simulink model "ESCHighLevelSim"  (R2021b)
settings: Solver=FixedStepDiscrete  StartTime=0.0  StopTime=15  FixedStep=0.008  RelTol=1e-3
InitFcn:
  | ts = 0.008
  | ESCHighLevelInit
values from neighbouring files (symbols this model uses):
  AbsActSpdThre = 10/3.6    (= 2.77777777778)    [ESCHighLevelInit.m]
  AbsBrkChkThre = 0.8    [ESCHighLevelInit.m]
  AbsCriDelay = 4    [ESCHighLevelInit.m]
  AbsLockJudgeThre = 0.006    [ESCHighLevelInit.m]
  AbsLockSlipThre1 = 0.05    [ESCHighLevelInit.m]
  AbsLockSlipThre2 = 0.15    [ESCHighLevelInit.m]
  AbsSpdEstRelayT = 40    [ESCHighLevelInit.m]
  FrontAngleDeadZone = 0.5*3.14/180    (= 0.00872222222222)    [ESCHighLevelInit.m]
  VehParaD = 1.958    [ESCHighLevelInit.m]
  VehParaL = 4.39    [ESCHighLevelInit.m]
  VehParaR = 0.376    [ESCHighLevelInit.m]
undefined symbols (not defined in the file or in its folder): Discrete, Time, VehR
libraries: dspstat3 x7, simulink x5, ctrlSharedLib x1
settings Model: Creator=Huiqian  LastModifiedBy=Huiqian
settings OptimizationCC: DefaultParameterBehavior=Inlined  UseDivisionForNetSlopeComputation=on  GainParamInheritBuiltInType=on  UseFloatMulNetSlope=on  InlineInvariantSignals=on  PassReuseOutputArgsAs=Individual arguments  ZeroExternalMemoryAtStartup=off  ZeroInternalMemoryAtStartup=off  NoFixptDivByZeroProtection=on  EfficientFloat2IntCast=on  LifeSpan=1  OptimizeBlockOrder=speed  DifferentSizesBufferReuse=on  EfficientTunableParamExpr=on
settings DebuggingCC: ParameterTunabilityLossMsg=error
settings HardwareCC: ProdBitPerPointer=32  ProdBitPerSizeT=32  ProdBitPerPtrDiffT=32  ProdLargestAtomicInteger=Long  ProdLargestAtomicFloat=Double  ProdWordSize=32  ProdLongLongMode=on  ProdHWDeviceType=NXP->Cortex-M4
settings SFSimCC: MATLABDynamicMemAlloc=off
settings RTWCC: Description=Embedded Coder  SystemTargetFile=ert.tlc  TemplateMakefile=ert_default_tmf  GenerateReport=on  LaunchReport=on
settings CodeAppCC: ForceParamTrailComments=on  IgnoreCustomStorageClasses=off  OperatorAnnotations=on  SimulinkDataObjDesc=on  SFDataObjDesc=on  CustomSymbolStrGlobalVar=rt$N$M  CustomSymbolStrType=$N$M  CustomSymbolStrFcn=$N$M$F  CustomSymbolStrMacro=$N$M  InsertBlockDesc=on
settings ERTTargetCC: TargetLangStandard=C99 (ISO)  GenerateSampleERTMain=on  IncludeMdlTerminateFcn=off  CombineSignalStateStructs=on  CodeInterfacePackaging=Reusable function  SupportComplex=off  SupportContinuousTime=on  SupportNonInlinedSFcns=on  InlinedParameterPlacement=NonHierarchical  ERTCustomFileTemplate=example_file_process.tlc

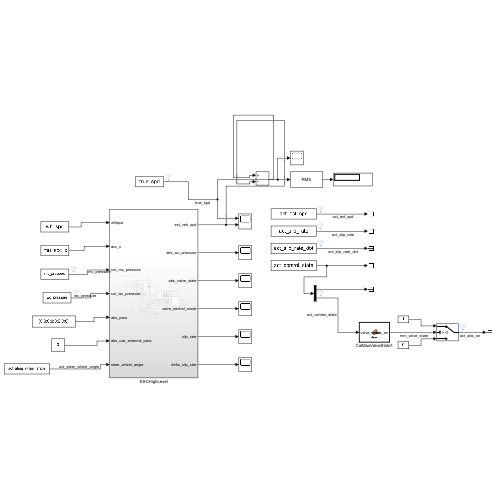
[thumbnail: Simulink's stored preview of the top-level diagram]
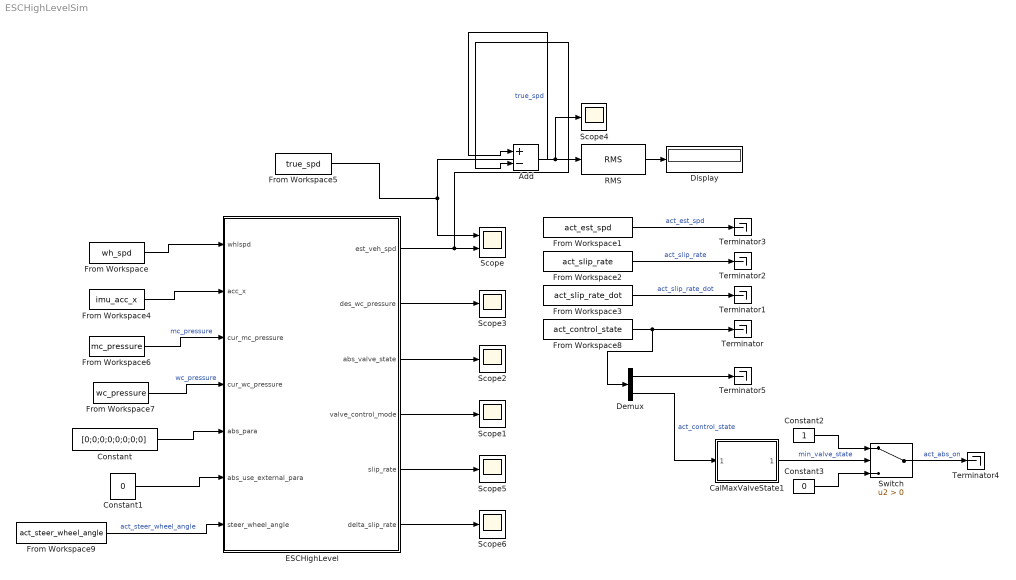
== system ESCHighLevelSim ==
  Add : Sum  Inputs=+-
  CalMaxValveState1 : MATLAB Function  TreatAsAtomicUnit=on
  Constant : Constant  Value=[0;0;0;0;0;0;0;0]  OutDataTypeStr=single
  Constant1 : Constant  Value=0  OutDataTypeStr=int32
  Constant2 : Constant  OutDataTypeStr=boolean
  Constant3 : Constant  Value=0  OutDataTypeStr=fixdt(1,16)
  Demux : Demux  Outputs=[2,4]
  Display : Display
  ESCHighLevel : Subsystem
  From Workspace : FromWorkspace  VariableName=wh_spd
  From Workspace1 : FromWorkspace  VariableName=act_est_spd
  From Workspace2 : FromWorkspace  VariableName=act_slip_rate
  From Workspace3 : FromWorkspace  VariableName=act_slip_rate_dot
  From Workspace4 : FromWorkspace  VariableName=imu_acc_x
  From Workspace5 : FromWorkspace  VariableName=true_spd
  From Workspace6 : FromWorkspace  VariableName=mc_pressure
  From Workspace7 : FromWorkspace  VariableName=wc_pressure
  From Workspace8 : FromWorkspace  VariableName=act_control_state
  From Workspace9 : FromWorkspace  VariableName=act_steer_wheel_angle
  RMS : dspstat3/RMS  run=off  directionMode=Each column  dimension=1  InputProcessing=Columns as channels (frame based)  reset_popup=None
  Scope : Scope  NumInputPorts=2
  Scope{1..6} (6 alike) : Scope
  Switch : Switch  Criteria=u2 > Threshold
  Terminator{,1..5} (6 alike) : Terminator
  wires:
  From Workspace/1 -> ESCHighLevel/1(whlspd)
  From Workspace6/1 -> ESCHighLevel/3(cur_mc_pressure)  "mc_pressure"
  ESCHighLevel/1(est_veh_spd) -> Add/2, Scope/2
  ESCHighLevel/2(des_wc_pressure) -> Scope3/1
  From Workspace7/1 -> ESCHighLevel/4(cur_wc_pressure)  "wc_pressure"
  From Workspace5/1 -> Scope/1, Add/1  "true_spd"
  Add/1 -> Scope4/1, RMS/1
  RMS/1 -> Display/1
  From Workspace4/1 -> ESCHighLevel/2(acc_x)
  ESCHighLevel/4(valve_control_mode) -> Scope1/1
  ESCHighLevel/3(abs_valve_state) -> Scope2/1
  Constant/1 -> ESCHighLevel/5(abs_para)
  Constant1/1 -> ESCHighLevel/6(abs_use_external_para)
  ESCHighLevel/5(slip_rate) -> Scope5/1
  ESCHighLevel/6(delta_slip_rate) -> Scope6/1
  From Workspace8/1 -> Demux/1, Terminator/1
  From Workspace3/1 -> Terminator1/1  "act_slip_rate_dot"
  From Workspace1/1 -> Terminator3/1  "act_est_spd"
  From Workspace2/1 -> Terminator2/1  "act_slip_rate"
  Switch/1 -> Terminator4/1  "act_abs_on"
  CalMaxValveState1/1(abs_on) -> Switch/2  "min_valve_state"
  Constant3/1 -> Switch/3
  Constant2/1 -> Switch/1
  Demux/1 -> Terminator5/1
  Demux/2 -> CalMaxValveState1/1(valve_state)  "act_control_state"
  From Workspace9/1 -> ESCHighLevel/7(steer_wheel_angle)  "act_steer_wheel_angle"

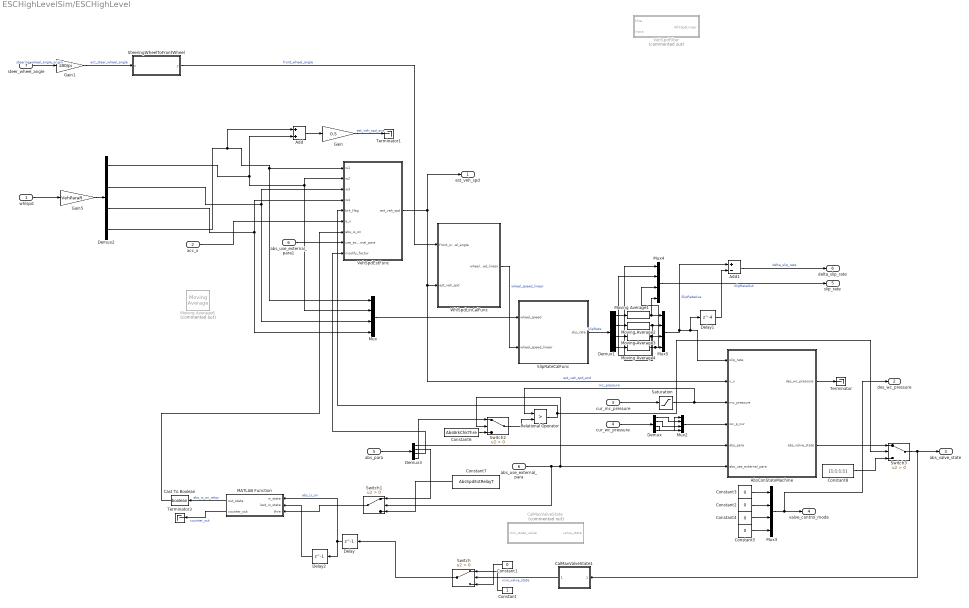
== system ESCHighLevelSim/ESCHighLevel ==
  whlspd : Inport  OutDataTypeStr=double  Unit=rad/s  PortDimensions=4
  acc_x : Inport  Port=2  OutDataTypeStr=double  Unit=m/s^2  PortDimensions=1
  cur_mc_pressure : Inport  Port=3  OutDataTypeStr=double  PortDimensions=1
  cur_wc_pressure : Inport  Port=4  OutDataTypeStr=double  PortDimensions=4
  abs_para : Inport  Port=5  OutDataTypeStr=single  PortDimensions=8
  abs_use_external_para : Inport  Port=6  OutDataTypeStr=int32  PortDimensions=1
  steer_wheel_angle : Inport  Port=7
  AbsConStateMachine : Subsystem  SystemSampleTime=0.01
      settings: MinAlgLoopOccurrences=on  RTWFcnNameOpts=Use subsystem name  RTWFileNameOpts=Use subsystem name
  Add : Sum
  Add1 : Sum  Inputs=+-
  CalMaxValveState : MATLAB Function  Commented=on  TreatAsAtomicUnit=on
  CalMaxValveState1 : MATLAB Function  TreatAsAtomicUnit=on
  Cast To Boolean : DataTypeConversion  OutDataTypeStr=boolean
  Constant : Constant  OutDataTypeStr=boolean
  Constant1 : Constant  Value=0  OutDataTypeStr=fixdt(1,16)
  Constant{2..5} (4 alike) : Constant  Value=0  OutDataTypeStr=int32
  Constant6 : Constant  Value=AbsBrkChkThre
  Constant7 : Constant  Value=AbsSpdEstRelayT
  Constant8 : Constant  Value=[1;1;1;1]
  Delay : Delay  DelayLength=1
  Delay1 : Delay  DelayLength=4
  Delay2 : Delay  DelayLength=1
  Demux : Demux
  Demux1 : Demux
  Demux2 : Demux
  Demux3 : Demux  Outputs=[5,1,1,1]
  Gain : Gain  Gain=0.5
  Gain1 : Gain  Gain=180/pi
  Gain5 : Gain  Gain=VehParaR
  MATLAB Function : MATLAB Function  TreatAsAtomicUnit=on
  Moving Average{1..4} (4 alike) : dspstat3/Moving Average  Method=Sliding window  ForgettingFactorPort=off  SpecifyWindowLength=on  WindowLength=3  ForgettingFactor=0.9  SimulateUsing=Code generation
  Moving Average6 : dspstat3/Moving Average  Commented=on  Method=Sliding window  ForgettingFactorPort=off  SpecifyWindowLength=on  WindowLength=5  ForgettingFactor=0.9  SimulateUsing=Code generation
  Mux{,2..5} (5 alike) : Mux
  Relational Operator : RelationalOperator  Operator=>  OutDataTypeStr=boolean  RndMeth=Simplest
  Saturation : Saturate  UpperLimit=10
  SlipRateCalFunc : Subsystem  TreatAsAtomicUnit=on
      settings: RTWFcnNameOpts=Use subsystem name  RTWFileNameOpts=Use subsystem name
  SteeringWheelToFrontWheel : MATLAB Function  TreatAsAtomicUnit=on
  Switch{,1..3} (4 alike) : Switch  Criteria=u2 > Threshold
  Terminator : Terminator
  Terminator1 : Terminator
  Terminator3 : Terminator
  VehSpdEstFunc : Subsystem  TreatAsAtomicUnit=on  SystemSampleTime=ts  RTWFcnName=VehSpdEstFunction  RTWFileName=VehSpdEstFunction
      settings: RTWFcnNameOpts=User specified  RTWFileNameOpts=User specified
  VehSpdFilter : Subsystem  Commented=on  TreatAsAtomicUnit=on
  WhlSpdLinCalFunc : Subsystem
  abs_use_external_para1 : InportShadow  Port=6  OutDataTypeStr=int32  PortDimensions=1
  est_veh_spd : Outport  OutDataTypeStr=double  Unit=m/s  PortDimensions=1
  des_wc_pressure : Outport  Port=2  PortDimensions=4
  abs_valve_state : Outport  Port=3  OutDataTypeStr=int32  PortDimensions=4
  valve_control_mode : Outport  Port=4  OutDataTypeStr=int32
  slip_rate : Outport  Port=5  OutDataTypeStr=double
  delta_slip_rate : Outport  Port=6  OutDataTypeStr=double
  wires:
  Demux3/4 -> Switch2/1
  Constant6/1 -> Switch2/3
  AbsConStateMachine/2(abs_valve_state) -> Switch3/1
  Switch3/1 -> abs_valve_state/1, CalMaxValveState1/1(valve_state)
  Constant8/1 -> Switch3/3
  Demux/3 -> Mux2/4
  Delay1/1 -> Add1/2
  Constant5/1 -> Mux3/4
  Demux/2 -> Mux2/3
  AbsConStateMachine/1(des_wc_pressure) -> Terminator/1
  Saturation/1 -> Relational Operator/1, AbsConStateMachine/3(mc_pressure)  "mc_pressure"
  Demux1/4 -> Moving Average4/1
  SlipRateCalFunc/1(slip_rate) -> Demux1/1  "SlipRate"
  Gain5/1 -> Demux2/1
  Switch1/1 -> MATLAB Function/3(thre)
  Demux1/1 -> Moving Average1/1
  Constant7/1 -> Switch1/3
  Demux3/2 -> Switch1/1
  Demux3/1 -> AbsConStateMachine/5(abs_para)
  Switch/1 -> Delay/1
  abs_para/1 -> Demux3/1
  Delay2/1 -> MATLAB Function/2(last_in_state)
  CalMaxValveState1/1(abs_on) -> Switch/2  "min_valve_state"
  Constant/1 -> Switch/1
  Add1/1 -> delta_slip_rate/1  "delta_slip_rate"
  cur_wc_pressure/1 -> Demux/1
  cur_mc_pressure/1 -> Saturation/1
  WhlSpdLinCalFunc/1(wheel_speed_linear) -> SlipRateCalFunc/2(wheel_speed_linear)  "wheel_speed_linear"
  Gain/1 -> Terminator1/1  "est_veh_spd_ave"
  MATLAB Function/2(counter_out) -> Terminator3/1  "counter_out"
  MATLAB Function/1(out_state) -> Cast To Boolean/1  "abs_is_on_relay"
  Moving Average2/1 -> Mux4/1, Mux5/2
  Mux/1 -> SlipRateCalFunc/1(wheel_speed)
  Switch2/1 -> Relational Operator/2
  Cast To Boolean/1 -> VehSpdEstFunc/7(abs_is_on)
  Demux3/3 -> VehSpdEstFunc/9(modify_factor)
  SteeringWheelToFrontWheel/1(y) -> WhlSpdLinCalFunc/1(front_wheel_angle)  "front_wheel_angle"
  Delay/1 -> Delay2/1, MATLAB Function/1(in_state)  "abs_is_on"
  steer_wheel_angle/1 -> Gain1/1  "steering_wheel_angle_origin"
  whlspd/1 -> Gain5/1
  Demux2/4 -> Add/1, Mux/1, VehSpdEstFunc/1(w1)
  Relational Operator/1 -> Switch3/2, VehSpdEstFunc/5(brk_flag)
  Demux1/3 -> Moving Average3/1
  Demux2/2 -> Mux/3, VehSpdEstFunc/3(w3)
  acc_x/1 -> VehSpdEstFunc/6(a_x)
  Demux2/1 -> Mux/2, VehSpdEstFunc/2(w2), Add/2
  abs_use_external_para/1 -> Switch1/2, Switch2/2, AbsConStateMachine/6(abs_use_external_para)
  Mux5/1 -> Add1/1, Delay1/1, AbsConStateMachine/1(slip_rate)  "SlipRateAve"
  Moving Average3/1 -> Mux5/3, Mux4/2
  Gain1/1 -> SteeringWheelToFrontWheel/1(x)  "act_steer_wheel_angle"
  Mux3/1 -> des_wc_pressure/1, valve_control_mode/1
  Demux/1 -> Mux2/2
  Constant1/1 -> Switch/3
  VehSpdEstFunc/1(est_veh_spd) -> est_veh_spd/1, WhlSpdLinCalFunc/2(est_veh_spd), AbsConStateMachine/2(v_x)  "est_veh_spd_end"
  Mux4/1 -> slip_rate/1  "SlipRateOut"
  Demux1/2 -> Moving Average2/1
  Constant2/1 -> Mux3/2
  Moving Average4/1 -> Mux4/3, Mux5/4
  Moving Average1/1 -> Mux4/4, Mux5/1
  Demux/4 -> Mux2/1
  Constant3/1 -> Mux3/1
  abs_use_external_para1/1 -> VehSpdEstFunc/8(use_external_para)
  Demux2/3 -> VehSpdEstFunc/4(w4), Mux/4
  Mux2/1 -> AbsConStateMachine/4(wc_p_cur)
  Constant4/1 -> Mux3/3
  Add/1 -> Gain/1

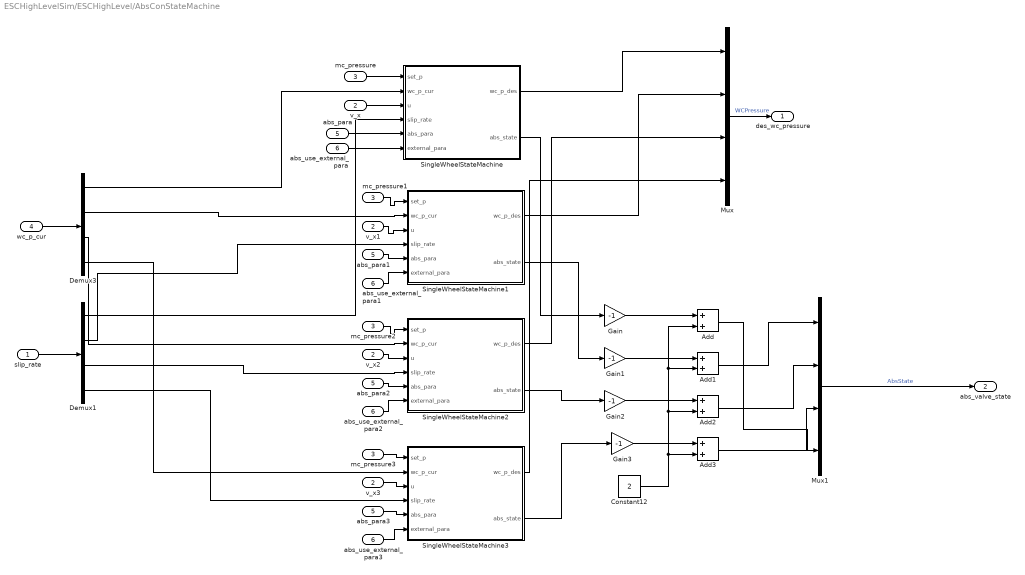
== system ESCHighLevelSim/ESCHighLevel/AbsConStateMachine ==
  slip_rate : Inport
  v_x : Inport  Port=2
  mc_pressure : Inport  Port=3
  wc_p_cur : Inport  Port=4
  abs_para : Inport  Port=5
  abs_use_external_para : Inport  Port=6  PortDimensions=1
  Add{,1..3} (4 alike) : Sum
  Constant12 : Constant  Value=2  OutDataTypeStr=int32
  Demux1 : Demux
  Demux3 : Demux
  Gain{,1..3} (4 alike) : Gain  Gain=-1  OutDataTypeStr=int32
  Mux : Mux
  Mux1 : Mux
  SingleWheelStateMachine : Subsystem  TreatAsAtomicUnit=on
  SingleWheelStateMachine1 : Subsystem  TreatAsAtomicUnit=on
  SingleWheelStateMachine2 : Subsystem  TreatAsAtomicUnit=on
  SingleWheelStateMachine3 : Subsystem  TreatAsAtomicUnit=on
  abs_para1 : InportShadow  Port=5
  abs_para2 : InportShadow  Port=5
  abs_para3 : InportShadow  Port=5
  abs_use_external_para1 : InportShadow  Port=6  PortDimensions=1
  abs_use_external_para2 : InportShadow  Port=6  PortDimensions=1
  abs_use_external_para3 : InportShadow  Port=6  PortDimensions=1
  mc_pressure1 : InportShadow  Port=3
  mc_pressure2 : InportShadow  Port=3
  mc_pressure3 : InportShadow  Port=3
  v_x1 : InportShadow  Port=2
  v_x2 : InportShadow  Port=2
  v_x3 : InportShadow  Port=2
  des_wc_pressure : Outport
  abs_valve_state : Outport  Port=2
  wires:
  Mux1/1 -> abs_valve_state/1  "AbsState"
  wc_p_cur/1 -> Demux3/1
  Mux/1 -> des_wc_pressure/1  "WCPressure"
  mc_pressure/1 -> SingleWheelStateMachine/1(set_p)
  slip_rate/1 -> Demux1/1
  Gain/1 -> Add/1
  Gain1/1 -> Add1/1
  Gain2/1 -> Add2/1
  Gain3/1 -> Add3/1
  Constant12/1 -> Add3/2, Add2/2, Add1/2, Add/2
  Add1/1 -> Mux1/1
  Add2/1 -> Mux1/2
  Add3/1 -> Mux1/3
  Add/1 -> Mux1/4
  Demux3/1 -> SingleWheelStateMachine/2(wc_p_cur)
  v_x/1 -> SingleWheelStateMachine/3(u)
  Demux1/1 -> SingleWheelStateMachine/4(slip_rate)
  abs_use_external_para/1 -> SingleWheelStateMachine/6(external_para)
  abs_para/1 -> SingleWheelStateMachine/5(abs_para)
  Demux3/2 -> SingleWheelStateMachine1/2(wc_p_cur)
  Demux1/2 -> SingleWheelStateMachine1/4(slip_rate)
  mc_pressure1/1 -> SingleWheelStateMachine1/1(set_p)
  v_x1/1 -> SingleWheelStateMachine1/3(u)
  abs_para1/1 -> SingleWheelStateMachine1/5(abs_para)
  abs_use_external_para1/1 -> SingleWheelStateMachine1/6(external_para)
  mc_pressure2/1 -> SingleWheelStateMachine2/1(set_p)
  mc_pressure3/1 -> SingleWheelStateMachine3/1(set_p)
  v_x2/1 -> SingleWheelStateMachine2/3(u)
  v_x3/1 -> SingleWheelStateMachine3/3(u)
  Demux3/3 -> SingleWheelStateMachine2/2(wc_p_cur)
  Demux3/4 -> SingleWheelStateMachine3/2(wc_p_cur)
  abs_para2/1 -> SingleWheelStateMachine2/5(abs_para)
  abs_para3/1 -> SingleWheelStateMachine3/5(abs_para)
  Demux1/3 -> SingleWheelStateMachine2/4(slip_rate)
  Demux1/4 -> SingleWheelStateMachine3/4(slip_rate)
  abs_use_external_para2/1 -> SingleWheelStateMachine2/6(external_para)
  abs_use_external_para3/1 -> SingleWheelStateMachine3/6(external_para)
  SingleWheelStateMachine3/2(abs_state) -> Gain3/1
  SingleWheelStateMachine2/2(abs_state) -> Gain2/1
  SingleWheelStateMachine1/2(abs_state) -> Gain1/1
  SingleWheelStateMachine/2(abs_state) -> Gain/1
  SingleWheelStateMachine3/1(wc_p_des) -> Mux/4
  SingleWheelStateMachine2/1(wc_p_des) -> Mux/3
  SingleWheelStateMachine1/1(wc_p_des) -> Mux/2
  SingleWheelStateMachine/1(wc_p_des) -> Mux/1

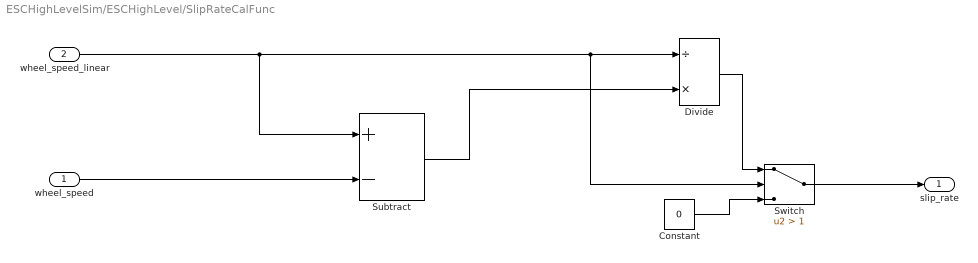
== system ESCHighLevelSim/ESCHighLevel/SlipRateCalFunc ==
  wheel_speed : Inport
  wheel_speed_linear : Inport  Port=2
  Constant : Constant  Value=0
  Divide : Product  Inputs=/*
  Subtract : Sum  Inputs=+-
  Switch : Switch  Criteria=u2 > Threshold  Threshold=1
  slip_rate : Outport
  wires:
  Subtract/1 -> Divide/2
  wheel_speed_linear/1 -> Subtract/1, Switch/2, Divide/1
  wheel_speed/1 -> Subtract/2
  Constant/1 -> Switch/3
  Divide/1 -> Switch/1
  Switch/1 -> slip_rate/1

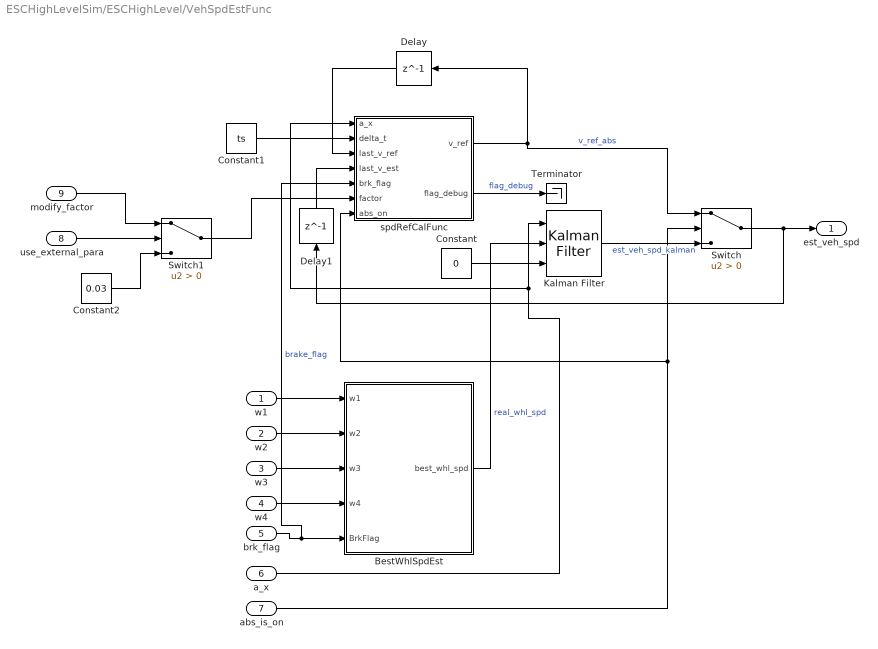
== system ESCHighLevelSim/ESCHighLevel/VehSpdEstFunc ==
  w1 : Inport  OutDataTypeStr=double
  w2 : Inport  Port=2  OutDataTypeStr=double
  w3 : Inport  Port=3  OutDataTypeStr=double
  w4 : Inport  Port=4  OutDataTypeStr=double
  brk_flag : Inport  Port=5  OutDataTypeStr=boolean
  a_x : Inport  Port=6  OutDataTypeStr=double
  abs_is_on : Inport  Port=7  OutDataTypeStr=boolean
  use_external_para : Inport  Port=8
  modify_factor : Inport  Port=9
  BestWhlSpdEst : MATLAB Function  TreatAsAtomicUnit=on
  Constant : Constant  Value=0
  Constant1 : Constant  Value=ts
  Constant2 : Constant  Value=0.03
  Delay : Delay  DelayLength=1
  Delay1 : Delay  DelayLength=1
  Kalman Filter : ctrlSharedLib/Kalman Filter  TimeDomain=Discrete-Time  UseCurrentEstimator=on  ModelSource=Individual A, B, C, D matrices  ModelSourceVariable=ss(0.95,1,1,0,1)  A=1  B=ts  C=1  D=0  NumberOfStates=1  NumberOfInputs=1  NumberOfOutputs=1  InitialEstimateSource=Input port  X0=0  P0=10  UseK=off  UseGH=off  NumberOfProcessNoiseInputs=1  G=1  TimeInvariantG=on  H=0  TimeInvariantH=on  Q=0.2  TimeInvariantQ=on  R=0.1  TimeInvariantR=on  N=0  TimeInvariantN=on  AddInputPort=on  AddEnablePort=off  OutputEstimatedY=off  OutputP=off  Ts=-1
  Switch : Switch  Criteria=u2 > Threshold
  Switch1 : Switch  Criteria=u2 > Threshold
  Terminator : Terminator
  spdRefCalFunc : MATLAB Function  TreatAsAtomicUnit=on
  est_veh_spd : Outport  OutDataTypeStr=double
  wires:
  Switch/1 -> Delay1/1, est_veh_spd/1
  abs_is_on/1 -> spdRefCalFunc/7(abs_on), Switch/2
  w3/1 -> BestWhlSpdEst/3(w3)
  w4/1 -> BestWhlSpdEst/4(w4)
  w2/1 -> BestWhlSpdEst/2(w2)
  brk_flag/1 -> spdRefCalFunc/5(brk_flag), BestWhlSpdEst/5(BrkFlag)  "brake_flag"
  a_x/1 -> Kalman Filter/1, spdRefCalFunc/1(a_x)
  w1/1 -> BestWhlSpdEst/1(w1)
  BestWhlSpdEst/1(best_whl_spd) -> Kalman Filter/2  "real_whl_spd"
  Constant/1 -> Kalman Filter/3
  Kalman Filter/1 -> Switch/3  "est_veh_spd_kalman"
  Constant1/1 -> spdRefCalFunc/2(delta_t)
  spdRefCalFunc/1(v_ref) -> Delay/1, Switch/1  "v_ref_abs"
  Delay/1 -> spdRefCalFunc/3(last_v_ref)
  Delay1/1 -> spdRefCalFunc/4(last_v_est)
  spdRefCalFunc/2(flag_debug) -> Terminator/1  "flag_debug"
  use_external_para/1 -> Switch1/2
  Switch1/1 -> spdRefCalFunc/6(factor)
  Constant2/1 -> Switch1/3
  modify_factor/1 -> Switch1/1

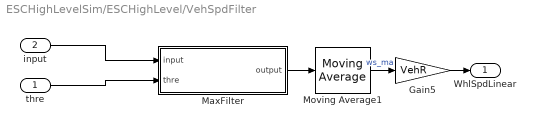
== system ESCHighLevelSim/ESCHighLevel/VehSpdFilter ==
  thre : Inport
  input : Inport  Port=2
  Gain5 : Gain  Gain=VehR
  MaxFilter : MATLAB Function  TreatAsAtomicUnit=on
  Moving Average1 : dspstat3/Moving Average  Method=Sliding window  ForgettingFactorPort=off  SpecifyWindowLength=on  WindowLength=5  ForgettingFactor=0.9  SimulateUsing=Code generation
  WhlSpdLinear : Outport
  wires:
  Moving Average1/1 -> Gain5/1  "ws_ma"
  Gain5/1 -> WhlSpdLinear/1
  MaxFilter/1(output) -> Moving Average1/1
  input/1 -> MaxFilter/1(input)
  thre/1 -> MaxFilter/2(thre)

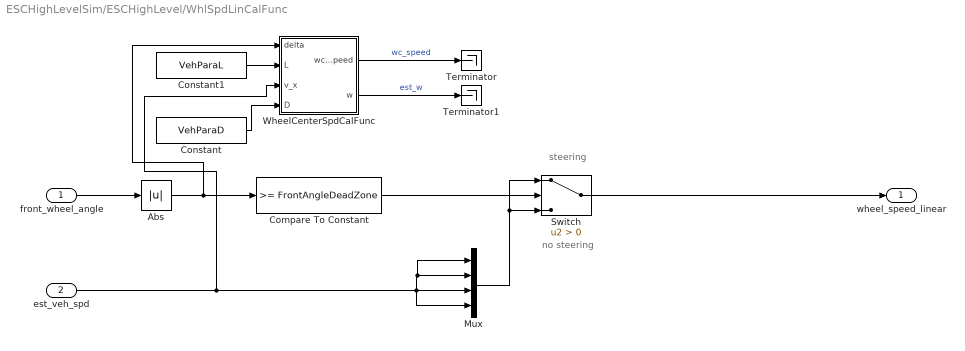
== system ESCHighLevelSim/ESCHighLevel/WhlSpdLinCalFunc ==
  note: no steering
  note: steering
  front_wheel_angle : Inport
  est_veh_spd : Inport  Port=2
  Abs : Abs
  Compare To Constant : simulink/Logic and Bit Operations/Compare To Constant  relop=>=  const=FrontAngleDeadZone  OutDataTypeStr=boolean
  Constant : Constant  Value=VehParaD
  Constant1 : Constant  Value=VehParaL
  Mux : Mux
  Switch : Switch  Criteria=u2 > Threshold
  Terminator : Terminator
  Terminator1 : Terminator
  WheelCenterSpdCalFunc : MATLAB Function  TreatAsAtomicUnit=on
  wheel_speed_linear : Outport
  wires:
  front_wheel_angle/1 -> Abs/1
  Abs/1 -> WheelCenterSpdCalFunc/1(delta), Compare To Constant/1
  Compare To Constant/1 -> Switch/2
  Switch/1 -> wheel_speed_linear/1
  est_veh_spd/1 -> WheelCenterSpdCalFunc/3(v_x), Mux/1, Mux/2, Mux/4, Mux/3
  Mux/1 -> Switch/1, Switch/3
  Constant/1 -> WheelCenterSpdCalFunc/4(D)
  Constant1/1 -> WheelCenterSpdCalFunc/2(L)
  WheelCenterSpdCalFunc/1(wc_speed) -> Terminator/1  "wc_speed"
  WheelCenterSpdCalFunc/2(w) -> Terminator1/1  "est_w"

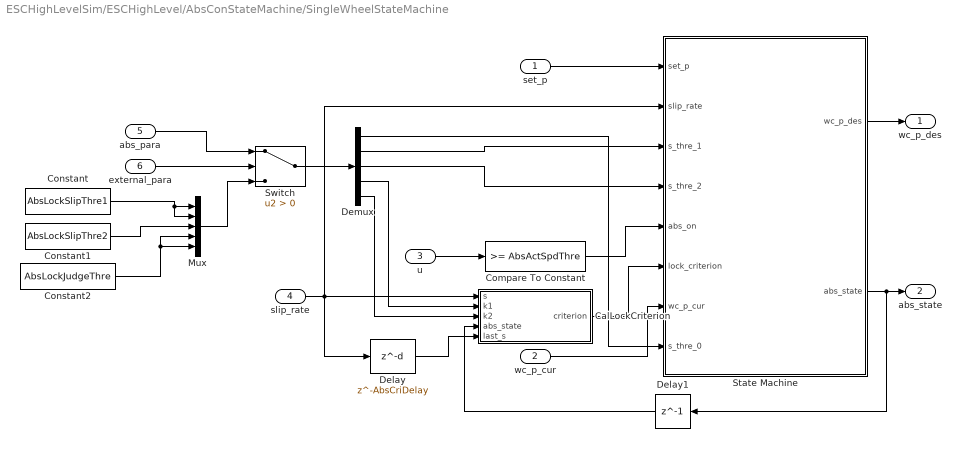
== system ESCHighLevelSim/ESCHighLevel/AbsConStateMachine/SingleWheelStateMachine ==
  set_p : Inport
  wc_p_cur : Inport  Port=2
  u : Inport  Port=3
  slip_rate : Inport  Port=4
  abs_para : Inport  Port=5
  external_para : Inport  Port=6
  CalLockCriterion : MATLAB Function  TreatAsAtomicUnit=on
  Compare To Constant : simulink/Logic and Bit Operations/Compare To Constant  relop=>=  const=AbsActSpdThre  OutDataTypeStr=boolean
  Constant : Constant  Value=AbsLockSlipThre1
  Constant1 : Constant  Value=AbsLockSlipThre2
  Constant2 : Constant  Value=AbsLockJudgeThre
  Delay : Delay  DelayLength=AbsCriDelay  InitialCondition=0
  Delay1 : Delay  DelayLength=1
  Demux : Demux  Outputs=5
  Mux : Mux  Inputs=5
  State Machine : Stateflow chart  TreatAsAtomicUnit=on
  Switch : Switch  Criteria=u2 > Threshold
  wc_p_des : Outport
  abs_state : Outport  Port=2  OutDataTypeStr=int32
  wires:
  Demux/3 -> State Machine/4(s_thre_2)
  u/1 -> Compare To Constant/1
  State Machine/2(abs_state) -> Delay1/1, abs_state/1
  Demux/2 -> State Machine/3(s_thre_1)
  set_p/1 -> State Machine/1(set_p)
  State Machine/1(wc_p_des) -> wc_p_des/1
  wc_p_cur/1 -> State Machine/7(wc_p_cur)
  Compare To Constant/1 -> State Machine/5(abs_on)
  Demux/4 -> CalLockCriterion/2(k1)
  Delay/1 -> CalLockCriterion/5(last_s)
  CalLockCriterion/1(criterion) -> State Machine/6(lock_criterion)
  slip_rate/1 -> Delay/1, CalLockCriterion/1(s), State Machine/2(slip_rate)
  Demux/1 -> State Machine/8(s_thre_0)
  external_para/1 -> Switch/2
  abs_para/1 -> Switch/1
  Switch/1 -> Demux/1
  Mux/1 -> Switch/3
  Constant2/1 -> Mux/5, Mux/4
  Constant/1 -> Mux/2, Mux/1
  Constant1/1 -> Mux/3
  Demux/5 -> CalLockCriterion/3(k2)
  Delay1/1 -> CalLockCriterion/4(abs_state)

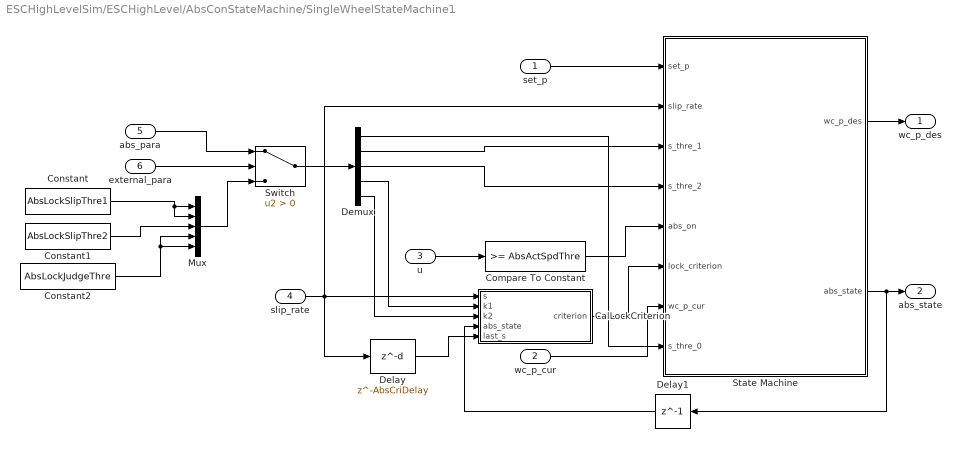
== system ESCHighLevelSim/ESCHighLevel/AbsConStateMachine/SingleWheelStateMachine1 ==
  set_p : Inport
  wc_p_cur : Inport  Port=2
  u : Inport  Port=3
  slip_rate : Inport  Port=4
  abs_para : Inport  Port=5
  external_para : Inport  Port=6
  CalLockCriterion : MATLAB Function  TreatAsAtomicUnit=on
  Compare To Constant : simulink/Logic and Bit Operations/Compare To Constant  relop=>=  const=AbsActSpdThre  OutDataTypeStr=boolean
  Constant : Constant  Value=AbsLockSlipThre1
  Constant1 : Constant  Value=AbsLockSlipThre2
  Constant2 : Constant  Value=AbsLockJudgeThre
  Delay : Delay  DelayLength=AbsCriDelay  InitialCondition=0
  Delay1 : Delay  DelayLength=1
  Demux : Demux  Outputs=5
  Mux : Mux  Inputs=5
  State Machine : Stateflow chart  TreatAsAtomicUnit=on
  Switch : Switch  Criteria=u2 > Threshold
  wc_p_des : Outport
  abs_state : Outport  Port=2  OutDataTypeStr=int32
  wires:
  Delay1/1 -> CalLockCriterion/4(abs_state)
  Demux/5 -> CalLockCriterion/3(k2)
  Constant1/1 -> Mux/3
  Constant/1 -> Mux/1, Mux/2
  Constant2/1 -> Mux/4, Mux/5
  Mux/1 -> Switch/3
  Switch/1 -> Demux/1
  abs_para/1 -> Switch/1
  external_para/1 -> Switch/2
  Demux/1 -> State Machine/8(s_thre_0)
  slip_rate/1 -> State Machine/2(slip_rate), CalLockCriterion/1(s), Delay/1
  CalLockCriterion/1(criterion) -> State Machine/6(lock_criterion)
  Delay/1 -> CalLockCriterion/5(last_s)
  Demux/4 -> CalLockCriterion/2(k1)
  Compare To Constant/1 -> State Machine/5(abs_on)
  wc_p_cur/1 -> State Machine/7(wc_p_cur)
  State Machine/1(wc_p_des) -> wc_p_des/1
  set_p/1 -> State Machine/1(set_p)
  Demux/2 -> State Machine/3(s_thre_1)
  State Machine/2(abs_state) -> abs_state/1, Delay1/1
  u/1 -> Compare To Constant/1
  Demux/3 -> State Machine/4(s_thre_2)

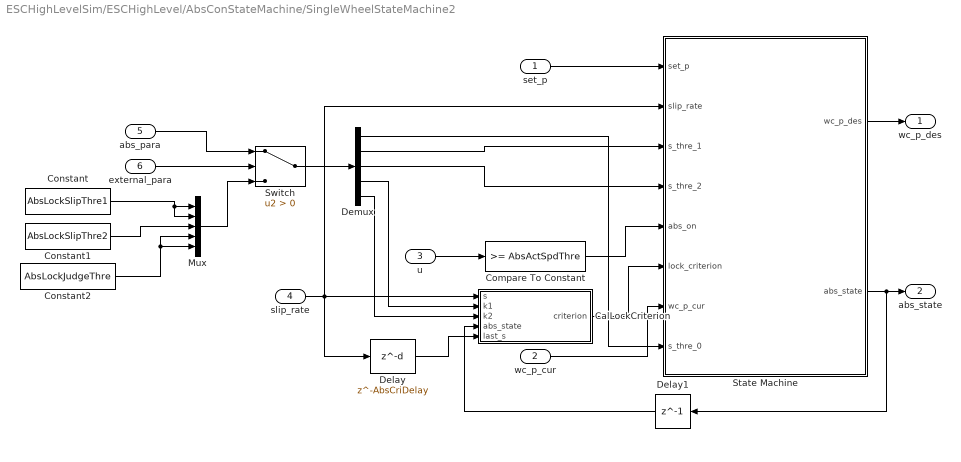
== system ESCHighLevelSim/ESCHighLevel/AbsConStateMachine/SingleWheelStateMachine2 ==
  set_p : Inport
  wc_p_cur : Inport  Port=2
  u : Inport  Port=3
  slip_rate : Inport  Port=4
  abs_para : Inport  Port=5
  external_para : Inport  Port=6
  CalLockCriterion : MATLAB Function  TreatAsAtomicUnit=on
  Compare To Constant : simulink/Logic and Bit Operations/Compare To Constant  relop=>=  const=AbsActSpdThre  OutDataTypeStr=boolean
  Constant : Constant  Value=AbsLockSlipThre1
  Constant1 : Constant  Value=AbsLockSlipThre2
  Constant2 : Constant  Value=AbsLockJudgeThre
  Delay : Delay  DelayLength=AbsCriDelay  InitialCondition=0
  Delay1 : Delay  DelayLength=1
  Demux : Demux  Outputs=5
  Mux : Mux  Inputs=5
  State Machine : Stateflow chart  TreatAsAtomicUnit=on
  Switch : Switch  Criteria=u2 > Threshold
  wc_p_des : Outport
  abs_state : Outport  Port=2  OutDataTypeStr=int32
  wires:
  Demux/3 -> State Machine/4(s_thre_2)
  u/1 -> Compare To Constant/1
  State Machine/2(abs_state) -> Delay1/1, abs_state/1
  Demux/2 -> State Machine/3(s_thre_1)
  set_p/1 -> State Machine/1(set_p)
  State Machine/1(wc_p_des) -> wc_p_des/1
  wc_p_cur/1 -> State Machine/7(wc_p_cur)
  Compare To Constant/1 -> State Machine/5(abs_on)
  Demux/4 -> CalLockCriterion/2(k1)
  Delay/1 -> CalLockCriterion/5(last_s)
  CalLockCriterion/1(criterion) -> State Machine/6(lock_criterion)
  slip_rate/1 -> Delay/1, CalLockCriterion/1(s), State Machine/2(slip_rate)
  Demux/1 -> State Machine/8(s_thre_0)
  external_para/1 -> Switch/2
  abs_para/1 -> Switch/1
  Switch/1 -> Demux/1
  Mux/1 -> Switch/3
  Constant2/1 -> Mux/5, Mux/4
  Constant/1 -> Mux/2, Mux/1
  Constant1/1 -> Mux/3
  Demux/5 -> CalLockCriterion/3(k2)
  Delay1/1 -> CalLockCriterion/4(abs_state)

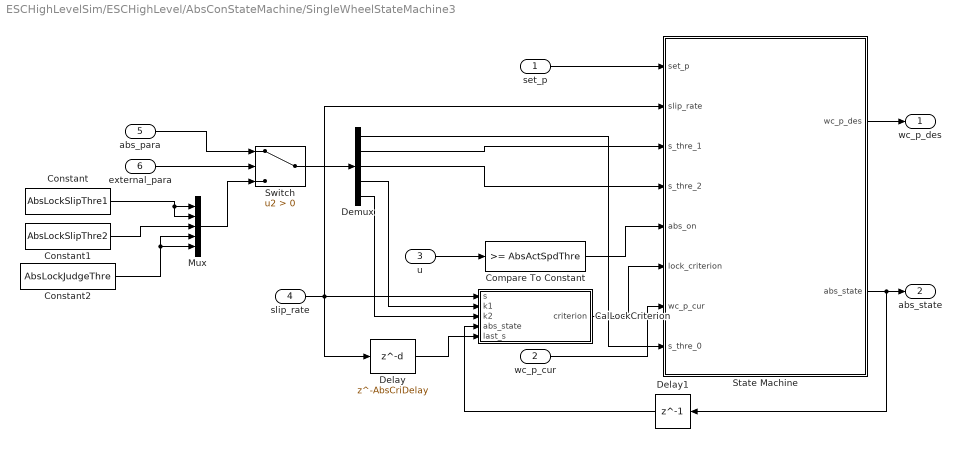
== system ESCHighLevelSim/ESCHighLevel/AbsConStateMachine/SingleWheelStateMachine3 ==
  set_p : Inport
  wc_p_cur : Inport  Port=2
  u : Inport  Port=3
  slip_rate : Inport  Port=4
  abs_para : Inport  Port=5
  external_para : Inport  Port=6
  CalLockCriterion : MATLAB Function  TreatAsAtomicUnit=on
  Compare To Constant : simulink/Logic and Bit Operations/Compare To Constant  relop=>=  const=AbsActSpdThre  OutDataTypeStr=boolean
  Constant : Constant  Value=AbsLockSlipThre1
  Constant1 : Constant  Value=AbsLockSlipThre2
  Constant2 : Constant  Value=AbsLockJudgeThre
  Delay : Delay  DelayLength=AbsCriDelay  InitialCondition=0
  Delay1 : Delay  DelayLength=1
  Demux : Demux  Outputs=5
  Mux : Mux  Inputs=5
  State Machine : Stateflow chart  TreatAsAtomicUnit=on
  Switch : Switch  Criteria=u2 > Threshold
  wc_p_des : Outport
  abs_state : Outport  Port=2  OutDataTypeStr=int32
  wires:
  Delay1/1 -> CalLockCriterion/4(abs_state)
  Demux/5 -> CalLockCriterion/3(k2)
  Constant1/1 -> Mux/3
  Constant/1 -> Mux/1, Mux/2
  Constant2/1 -> Mux/4, Mux/5
  Mux/1 -> Switch/3
  Switch/1 -> Demux/1
  abs_para/1 -> Switch/1
  external_para/1 -> Switch/2
  Demux/1 -> State Machine/8(s_thre_0)
  slip_rate/1 -> State Machine/2(slip_rate), CalLockCriterion/1(s), Delay/1
  CalLockCriterion/1(criterion) -> State Machine/6(lock_criterion)
  Delay/1 -> CalLockCriterion/5(last_s)
  Demux/4 -> CalLockCriterion/2(k1)
  Compare To Constant/1 -> State Machine/5(abs_on)
  wc_p_cur/1 -> State Machine/7(wc_p_cur)
  State Machine/1(wc_p_des) -> wc_p_des/1
  set_p/1 -> State Machine/1(set_p)
  Demux/2 -> State Machine/3(s_thre_1)
  State Machine/2(abs_state) -> abs_state/1, Delay1/1
  u/1 -> Compare To Constant/1
  Demux/3 -> State Machine/4(s_thre_2)

== stateflow chart ESCHighLevelSim/ESCHighLevel/AbsConStateMachine/SingleWheelStateMachine2/State Machine ==
  state Set_Pressure
    abs_state = 1;
    wc_p_tmp = set_p;
    wc_p_des = wc_p_tmp;
  state Keep_Pressure
    abs_state = 2;
    wc_p_des = wc_p_cur;
  state Reduce_Pressure
    abs_state = 3;
    wc_p_des = 0;
  (default) -> Set_Pressure
  Set_Pressure -> Keep_Pressure : [slip_rate>=s_thre_1&abs_on&lock_criterion>=0]
  Keep_Pressure -> Set_Pressure [order 2] : [slip_rate<s_thre_0]
  Reduce_Pressure -> Set_Pressure : [slip_rate<s_thre_0]
  Keep_Pressure -> Reduce_Pressure [order 1] : [slip_rate>=s_thre_2&lock_criterion>=0]
  data: set_p input double; slip_rate input double; wc_p_des output double; wc_p_tmp local double; abs_state output int32; s_thre_1 input; s_thre_2 input; abs_on input; lock_criterion input; wc_p_cur input; s_thre_0 input

== matlab function ESCHighLevelSim/ESCHighLevel/AbsConStateMachine/SingleWheelStateMachine3/CalLockCriterion ==
  data: criterion output; s input; k1 input; k2 input; abs_state input; last_s input
function criterion = fcn(s,k1,k2,abs_state,last_s)
% criterion = a_w + (s-1)*a_x -k*v;
dot_s = s - last_s;
k = k1;
if abs_state == 2
    k = k2;
end
% criterion = s-0.05;
criterion = dot_s - k;
end

== stateflow chart ESCHighLevelSim/ESCHighLevel/AbsConStateMachine/SingleWheelStateMachine3/State Machine ==
  state Set_Pressure
    abs_state = 1;
    wc_p_tmp = set_p;
    wc_p_des = wc_p_tmp;
  state Keep_Pressure
    abs_state = 2;
    wc_p_des = wc_p_cur;
  state Reduce_Pressure
    abs_state = 3;
    wc_p_des = 0;
  (default) -> Set_Pressure
  Set_Pressure -> Keep_Pressure : [slip_rate>=s_thre_1&abs_on&lock_criterion>=0]
  Keep_Pressure -> Set_Pressure [order 2] : [slip_rate<s_thre_0]
  Reduce_Pressure -> Set_Pressure : [slip_rate<s_thre_0]
  Keep_Pressure -> Reduce_Pressure [order 1] : [slip_rate>=s_thre_2&lock_criterion>=0]
  data: set_p input double; slip_rate input double; wc_p_des output double; wc_p_tmp local double; abs_state output int32; s_thre_1 input; s_thre_2 input; abs_on input; lock_criterion input; wc_p_cur input; s_thre_0 input

== matlab function ESCHighLevelSim/ESCHighLevel/SteeringWheelToFrontWheel ==
  data: x input; y output
function y = fcn(x)
%输入：方向盘转角 角度制 左负右正
%输出：前轮转角 弧度制 左正右负，与AYC的车辆坐标系统一
if(x>468) 
    x=468;
end
if(x<-468)
    x=-468;
end
y =8E-14*x^5-3E-11*x^4+2E-8*x^3-5E-6*x^2+0.0618*x-0.0278;
y=-y;
y=y/180*pi;

== matlab function ESCHighLevelSim/ESCHighLevel/VehSpdEstFunc/spdRefCalFunc ==
  data: a_x input; v_ref output; delta_t input; last_v_ref input; last_v_est input; brk_flag input; factor input; abs_on input; flag_debug output
function [v_ref,flag_debug] = fcn(a_x,delta_t,last_v_ref,last_v_est,brk_flag,factor,abs_on)
persistent modify_flag
if isempty(modify_flag)
    modify_flag = 0;
end
if brk_flag == 0
    modify_flag = 0;
end
if modify_flag == 0 && abs_on
    modify_flag = 1;
    v_ref = last_v_est*(1 + factor) + a_x * delta_t;
else
    v_ref = last_v_est + a_x * delta_t;
end
flag_debug = modify_flag;
end

== matlab function ESCHighLevelSim/ESCHighLevel/CalMaxValveState1 ==
  data: valve_state input; abs_on output
function abs_on = fcn(valve_state)
abs_on = 0;
for i = 1:4
    if valve_state(i)<0.5
        abs_on = 1;
    end
end
% if max(valve_state)<0.5
%     abs_on = 1;
% end
end

== matlab function ESCHighLevelSim/ESCHighLevel/WhlSpdLinCalFunc/WheelCenterSpdCalFunc ==
  data: delta input; wc_speed output; L input; v_x input; D input; w output
function [wc_speed,w] = fcn(delta,L,v_x,D)
R = L / tan(delta); 
w = v_x / R;
wc_speed = [w*sqrt((R-D/2)^2+L^2);w*sqrt((R+D/2)^2+L^2);w*(R-D/2);w*(R+D/2)];
% wc_speed = [0;0;0;0];
% wc_speed(1) = w*sqrt((R-D/2)^2+L^2);
% wc_speed(2) = w*sqrt((R+D/2)^2+L^2);
% wc_speed(3) = w*(R-D/2);
% wc_speed(4) = w*(R+D/2);
end

== matlab function ESCHighLevelSim/ESCHighLevel/MATLAB Function ==
  data: in_state input; out_state output; last_in_state input; thre input; counter_out output
function [out_state,counter_out] = fcn(in_state,last_in_state,thre)
persistent counter
if isempty(counter)
    counter = 0;
end

if in_state == 1
    out_state = 1;
    if counter < thre && counter > 0
        counter = counter + 1;
    else 
        counter = 0;
    end
else % in state == 0
   if last_in_state == 0
       if counter < thre && counter > 0
          out_state = 1;
          counter = counter + 1;
       else
          counter = 0;
          out_state = 0;
       end
   else % down side
       counter = 1;
       out_state = 1;
%        if counter < thre
%            out_state = 1;
%            counter = counter + 1;
%        else 
%            out_state = 0;
%        end
end
end
counter_out = counter;
end

== matlab function ESCHighLevelSim/CalMaxValveState1 ==
  data: valve_state input; abs_on output
function abs_on = fcn(valve_state)
abs_on = 0;
for i = 1:4
    if valve_state(i)<0.5
        abs_on = 1;
    end
end
% if max(valve_state)<0.5
%     abs_on = 1;
% end
end

== stateflow chart ESCHighLevelSim/ESCHighLevel/AbsConStateMachine/SingleWheelStateMachine/State Machine ==
  state Set_Pressure
    abs_state = 1;
    wc_p_tmp = set_p;
    wc_p_des = wc_p_tmp;
  state Keep_Pressure
    abs_state = 2;
    wc_p_des = wc_p_cur;
  state Reduce_Pressure
    abs_state = 3;
    wc_p_des = 0;
  (default) -> Set_Pressure
  Set_Pressure -> Keep_Pressure : [slip_rate>=s_thre_1&abs_on&lock_criterion>=0]
  Keep_Pressure -> Set_Pressure [order 2] : [slip_rate<s_thre_0]
  Reduce_Pressure -> Set_Pressure : [slip_rate<s_thre_0]
  Keep_Pressure -> Reduce_Pressure [order 1] : [slip_rate>=s_thre_2&lock_criterion>=0]
  data: set_p input double; slip_rate input double; wc_p_des output double; wc_p_tmp local double; abs_state output int32; s_thre_1 input; s_thre_2 input; abs_on input; lock_criterion input; wc_p_cur input; s_thre_0 input

== matlab function ESCHighLevelSim/ESCHighLevel/AbsConStateMachine/SingleWheelStateMachine/CalLockCriterion ==
  data: criterion output; s input; k1 input; k2 input; abs_state input; last_s input
function criterion = fcn(s,k1,k2,abs_state,last_s)
% criterion = a_w + (s-1)*a_x -k*v;
dot_s = s - last_s;
k = k1;
if abs_state == 2
    k = k2;
end
% criterion = s-0.05;
criterion = dot_s - k;
end

== matlab function ESCHighLevelSim/ESCHighLevel/CalMaxValveState ==
  data: valve_state input; min_state_value output
function min_state_value = fcn(valve_state)
min_state_value = min(valve_state);
end

== matlab function ESCHighLevelSim/ESCHighLevel/VehSpdEstFunc/BestWhlSpdEst ==
  data: w1 input; best_whl_spd output; w2 input; w3 input; w4 input; BrkFlag input
function best_whl_spd = fcn(w1,w2,w3,w4, BrkFlag)
    if BrkFlag % Brk on 
        best_whl_spd = max([w1,w2,w3,w4]);
    else
        best_whl_spd = (w1+w2)/2;
end

== matlab function ESCHighLevelSim/ESCHighLevel/VehSpdFilter/MaxFilter ==
  data: input input; output output; thre input
function output = fcn(input,thre)
    persistent data_store;
    N = 100;
    if isempty(data_store)
        data_store = zeros(N,1);
    end
    output = input;
    if input >= 3
        p = polyfit([0:1:N-1],data_store(1:N),1);
        est = p(1) * N + p(2);
        if abs(input - est) > thre
            output = est;
        end
    end
    data_store(1:N-1) = data_store(2:N);
    data_store(N) = output;
end

== matlab function ESCHighLevelSim/ESCHighLevel/AbsConStateMachine/SingleWheelStateMachine1/CalLockCriterion ==
  data: criterion output; s input; k1 input; k2 input; abs_state input; last_s input
function criterion = fcn(s,k1,k2,abs_state,last_s)
% criterion = a_w + (s-1)*a_x -k*v;
dot_s = s - last_s;
k = k1;
if abs_state == 2
    k = k2;
end
% criterion = s-0.05;
criterion = dot_s - k;
end

== stateflow chart ESCHighLevelSim/ESCHighLevel/AbsConStateMachine/SingleWheelStateMachine1/State Machine ==
  state Set_Pressure
    abs_state = 1;
    wc_p_tmp = set_p;
    wc_p_des = wc_p_tmp;
  state Keep_Pressure
    abs_state = 2;
    wc_p_des = wc_p_cur;
  state Reduce_Pressure
    abs_state = 3;
    wc_p_des = 0;
  (default) -> Set_Pressure
  Set_Pressure -> Keep_Pressure : [slip_rate>=s_thre_1&abs_on&lock_criterion>=0]
  Keep_Pressure -> Set_Pressure [order 2] : [slip_rate<s_thre_0]
  Reduce_Pressure -> Set_Pressure : [slip_rate<s_thre_0]
  Keep_Pressure -> Reduce_Pressure [order 1] : [slip_rate>=s_thre_2&lock_criterion>=0]
  data: set_p input double; slip_rate input double; wc_p_des output double; wc_p_tmp local double; abs_state output int32; s_thre_1 input; s_thre_2 input; abs_on input; lock_criterion input; wc_p_cur input; s_thre_0 input

== matlab function ESCHighLevelSim/ESCHighLevel/AbsConStateMachine/SingleWheelStateMachine2/CalLockCriterion ==
  data: criterion output; s input; k1 input; k2 input; abs_state input; last_s input
function criterion = fcn(s,k1,k2,abs_state,last_s)
% criterion = a_w + (s-1)*a_x -k*v;
dot_s = s - last_s;
k = k1;
if abs_state == 2
    k = k2;
end
% criterion = s-0.05;
criterion = dot_s - k;
end
